simulink library "lib_feed_foward_current_control"  (R2023a)
settings: Solver=VariableStepAuto  StartTime=0.0  StopTime=10.0  RelTol=1e-3
undefined symbols (not defined in the file): parDirCurrMaxVal, parDirIndcMaxVal, parElctSpdMaxVal, parPermMagFluxMaxVal, parPhsRstnMaxVal, parQdrtCurrMaxVal, parQdrtIndcMaxVal
libraries: lib_conversion x10, lib_dynamic_saturator x2
settings Model: Creator=cav2ofo  LastModifiedBy=lenovo
settings OptimizationCC: ReuseModelBlockBuffer=off

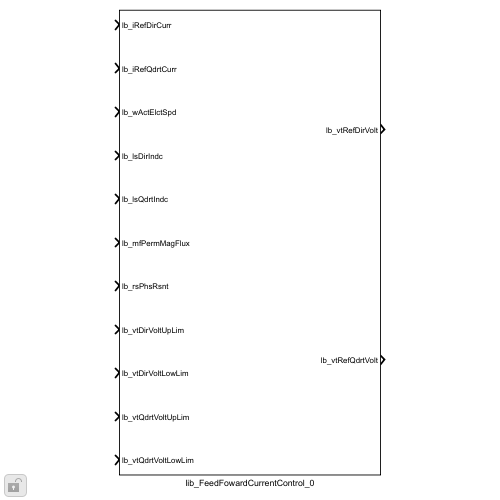
[thumbnail: Simulink's stored preview of the top-level diagram]
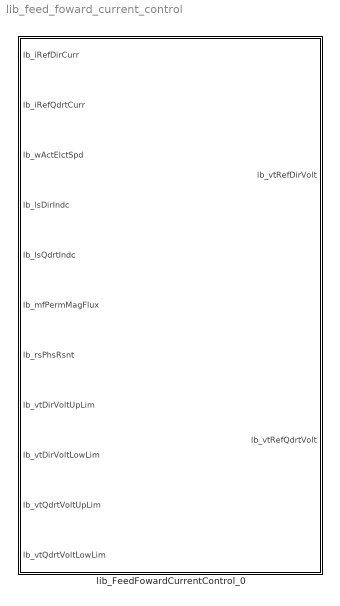
== system lib_feed_foward_current_control ==
  lib_FeedFowardCurrentControl_0 : Subsystem  mask{lb_parDirCurrMaxVal=parDirCurrMaxVal, lb_parDirCurrMinVal=-parDirCurrMaxVal, lb_parQdrtCurrMaxVal=parQdrtCurrMaxVal, lb_parQdrtCurrMinVal=-parQdrtCurrMaxVal, lb_parElctSpdMaxVal=parElctSpdMaxVal, lb_parElctSpdMinVal=-parElctSpdMaxVal, lb_parDirIndcMaxVal=parDirIndcMaxVal, lb_parQdrtIndcMaxVal=parQdrtIndcMaxVal, lb_parPhsRsntMaxVal=parPhsRstnMaxVal, lb_parPermMagFluxMaxVal=parPermMagFluxMaxVal, lb_parOutpDataType=fixdt(1,16,2^-9,0)}
      mask prompts: lb_parDirCurrMaxVal "Maximum direct current [A]:"; lb_parDirCurrMinVal "Minimum direct current [A]:"; lb_parQdrtCurrMaxVal "Maximum quadrature current [A]:"; lb_parQdrtCurrMinVal "Minimum quadrature current [A]:"; lb_parElctSpdMaxVal "Maximum electric speed [rad/s]:"; lb_parElctSpdMinVal "Minimum electric speed [rad/s]:"; lb_parDirIndcMaxVal "Maximum direct inductance [H]:"; lb_parQdrtIndcMaxVal "Maximum quadrature inductance [H]:"; lb_parPhsRsntMaxVal "Maximum phase resistance [Ohm]:"; lb_parPermMagFluxMaxVal "Maximum permanent magnet flux [Wb]:"; lb_parOutpDataType "Output data type:"
      mask init:
      | %% Req. XXX_ Define data type for product w*Lq
      | lb_parCnst1MaxVal = max(abs([lb_parElctSpdMaxVal,lb_parElctSpdMinVal]))*lb_parQdrtIndcMaxVal;
      | lb_parCnst1DataType = Simulink.NumericType;
      | lb_parCnst1DataType.DataTypeMode= 'Fixed-point: unspecified scaling';
      | lb_parCnst1DataType.Signedness = 'Signed';
      | lb_parCnst1DataType.WordLength = 16;
      | 
      | %% Req. XXX_ Define data type for product Id*Rs
      | lb_parCnst2MaxVal = max(abs([lb_parDirCurrMaxVal,lb_parDirCurrMinVal]))*lb_parPhsRsntMaxVal;
      | lb_parCnst2DataType = Simulink.NumericType;
      | lb_parCnst2DataType.DataTypeMode= 'Fixed-point: unspecified scaling';
      | lb_parCnst2DataType.Signedness = 'Signed';
      | lb_parCnst2DataType.WordLength = 16;
      | 
      | %% Req. XXX_ Define data type for product w*Lq*Iq
      | lb_parCnst3MaxVal = max(abs([lb_parQdrtCurrMaxVal,lb_parQdrtCurrMinVal]))*lb_parCnst1MaxVal;
      | lb_parCnst3DataType = Simulink.NumericType;
      | lb_parCnst3DataType.DataTypeMode= 'Fixed-point: unspecified scaling';
      | lb_parCnst3DataType.Signedness = 'Signed';
      | lb_parCnst3DataType.WordLength = 16;
      | 
      | %% Req. XXX_ Define data type for product Iq*Rs
      | lb_parCnst4MaxVal = max(abs([lb_parQdrtCurrMaxVal,lb_parQdrtCurrMinVal]))*lb_parPhsRsntMaxVal;
      | lb_parCnst4DataType = Simulink.NumericType;
      | lb_parCnst4DataType.DataTypeMode= 'Fixed-point: unspecified scaling';
      | lb_parCnst4DataType.Signedness = 'Signed';
      | lb_parCnst4DataType.WordLength = 16;
      | 
      | %% Req. XXX_ Define data type for product w*Ld
      | lb_parCnst5MaxVal = max(abs([lb_parElctSpdMaxVal,lb_parElctSpdMinVal]))*lb_parDirIndcMaxVal;
      | lb_parCnst5DataType = Simulink.NumericType;
      | lb_parCnst5DataType.DataTypeMode= 'Fixed-point: unspecified scaling';
      | lb_parCnst5DataType.Signedness = 'Signed';
      | lb_parCnst5DataType.WordLength = 16;
      | 
      | %% Req. XXX_ Define data type for product w*Ld*Id
      | lb_parCnst6MaxVal = max(abs([lb_parDirCurrMaxVal,lb_parDirCurrMinVal]))*lb_parCnst5MaxVal;
      | lb_parCnst6DataType = Simulink.NumericType;
      | lb_parCnst6DataType.DataTypeMode= 'Fixed-point: unspecified scaling';
      | lb_parCnst6DataType.Signedness = 'Signed';
      | lb_parCnst6DataType.WordLength = 16;
      | 
      | %% Req. XXX_ Define data type for product Iq*Rs+w*Ld*Id
      | lb_parCnst7MaxVal = lb_parCnst4MaxVal+lb_parCnst6MaxVal;
      | lb_parCnst7DataType = Simulink.NumericType;
      | lb_parCnst7DataType.DataTypeMode= 'Fixed-point: unspecified scaling';
      | lb_parCnst7DataType.Signedness = 'Signed';
      | lb_parCnst7DataType.WordLength = 16;
      | 
      | %% Req. XXX_ Define data type for product w*Ld
      | lb_parCnst8MaxVal = max(abs([lb_parElctSpdMaxVal,lb_parElctSpdMinVal]))*lb_parPermMagFluxMaxVal;
      | lb_parCnst8DataType = Simulink.NumericType;
      | lb_parCnst8DataType.DataTypeMode= 'Fixed-point: unspecified scaling';
      | lb_parCnst8DataType.Signedness = 'Signed';
      | lb_parCnst8DataType.WordLength = 16;
      mask TypeOptions lb_parOutpDataType: sss_DirectCurrentCoupling/lib_Conversion_1/lb_parDataType | sss_QuadratureCurrentCoupling/lib_Conversion_1/lb_parDataType
      mask DialogControl DescGroupVar Prompt: Current Coupling block
      mask DialogControl DescTextVar Prompt: This block computes the direct and quadrature voltage references.
      mask DialogControl modlPar Prompt: Parameter
      mask DialogControl Container3 Prompt: Data type

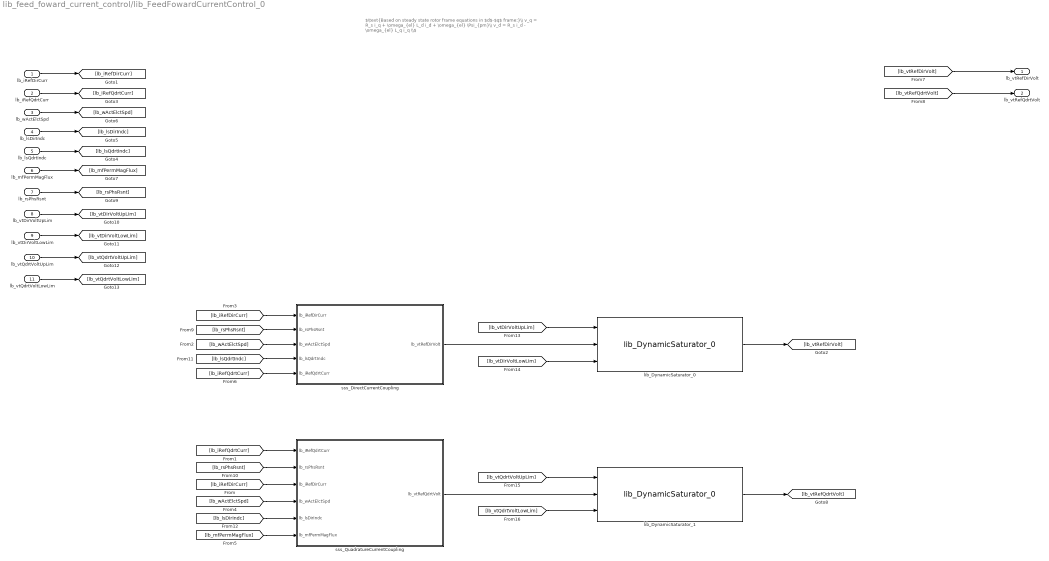
== system lib_feed_foward_current_control/lib_FeedFowardCurrentControl_0 ==
  note: $\text{Based on steady state rotor frame equations in $d$-$q$ frame:}\\ v_q = R_s i_q + \omega_{el} L_d i_d + \omega_{el} \Psi_{pm}\\ v_d = R_s i_d - \omega_{el} L_q i_q \\$
  lb_iRefDirCurr : Inport
  lb_iRefQdrtCurr : Inport  Port=2
  lb_wActElctSpd : Inport  Port=3
  lb_lsDirIndc : Inport  Port=4
  lb_lsQdrtIndc : Inport  Port=5
  lb_mfPermMagFlux : Inport  Port=6
  lb_rsPhsRsnt : Inport  Port=7
  lb_vtDirVoltUpLim : Inport  Port=8
  lb_vtDirVoltLowLim : Inport  Port=9
  lb_vtQdrtVoltUpLim : Inport  Port=10
  lb_vtQdrtVoltLowLim : Inport  Port=11
  lib_DynamicSaturator_0 : lib_dynamic_saturator/lib_DynamicSaturator_0
  lib_DynamicSaturator_1 : lib_dynamic_saturator/lib_DynamicSaturator_0
  sss_DirectCurrentCoupling : Subsystem
  sss_QuadratureCurrentCoupling : Subsystem
  lb_vtRefDirVolt : Outport
  lb_vtRefQdrtVolt : Outport  Port=2
  wires:
  [lb_wActElctSpd] -> sss_QuadratureCurrentCoupling/4(lb_wActElctSpd)
  lb_iRefDirCurr/1 -> [lb_iRefDirCurr]
  [lb_iRefDirCurr] -> sss_DirectCurrentCoupling/1(lb_iRefDirCurr)
  lb_lsDirIndc/1 -> [lb_lsDirIndc]
  [lb_vtRefQdrtVolt] -> lb_vtRefQdrtVolt/1
  [lb_wActElctSpd] -> sss_DirectCurrentCoupling/3(lb_wActElctSpd)
  lb_iRefQdrtCurr/1 -> [lb_iRefQdrtCurr]
  lb_lsQdrtIndc/1 -> [lb_lsQdrtIndc]
  [lb_mfPermMagFlux] -> sss_QuadratureCurrentCoupling/6(lb_mfPermMagFlux)
  [lb_iRefQdrtCurr] -> sss_DirectCurrentCoupling/5(lb_iRefQdrtCurr)
  lb_wActElctSpd/1 -> [lb_wActElctSpd]
  [lb_vtRefDirVolt] -> lb_vtRefDirVolt/1
  lb_mfPermMagFlux/1 -> [lb_mfPermMagFlux]
  [lb_iRefQdrtCurr] -> sss_QuadratureCurrentCoupling/1(lb_iRefQdrtCurr)
  [lb_iRefDirCurr] -> sss_QuadratureCurrentCoupling/3(lb_iRefDirCurr)
  lb_rsPhsRsnt/1 -> [lb_rsPhsRsnt]
  [lb_rsPhsRsnt] -> sss_DirectCurrentCoupling/2(lb_rsPhsRsnt)
  [lb_rsPhsRsnt] -> sss_QuadratureCurrentCoupling/2(lb_rsPhsRsnt)
  lib_DynamicSaturator_0/1 -> [lb_vtRefDirVolt]
  [lb_vtDirVoltUpLim] -> lib_DynamicSaturator_0/1
  [lb_vtDirVoltLowLim] -> lib_DynamicSaturator_0/3
  lib_DynamicSaturator_1/1 -> [lb_vtRefQdrtVolt]
  [lb_vtQdrtVoltLowLim] -> lib_DynamicSaturator_1/3
  [lb_vtQdrtVoltUpLim] -> lib_DynamicSaturator_1/1
  [lb_lsQdrtIndc] -> sss_DirectCurrentCoupling/4(lb_lsQdrtIndc)
  [lb_lsDirIndc] -> sss_QuadratureCurrentCoupling/5(lb_lsDirIndc)
  sss_DirectCurrentCoupling/1(lb_vtRefDirVolt) -> lib_DynamicSaturator_0/2
  sss_QuadratureCurrentCoupling/1(lb_vtRefQdrtVolt) -> lib_DynamicSaturator_1/2
  lb_vtDirVoltUpLim/1 -> [lb_vtDirVoltUpLim]
  lb_vtDirVoltLowLim/1 -> [lb_vtDirVoltLowLim]
  lb_vtQdrtVoltUpLim/1 -> [lb_vtQdrtVoltUpLim]
  lb_vtQdrtVoltLowLim/1 -> [lb_vtQdrtVoltLowLim]

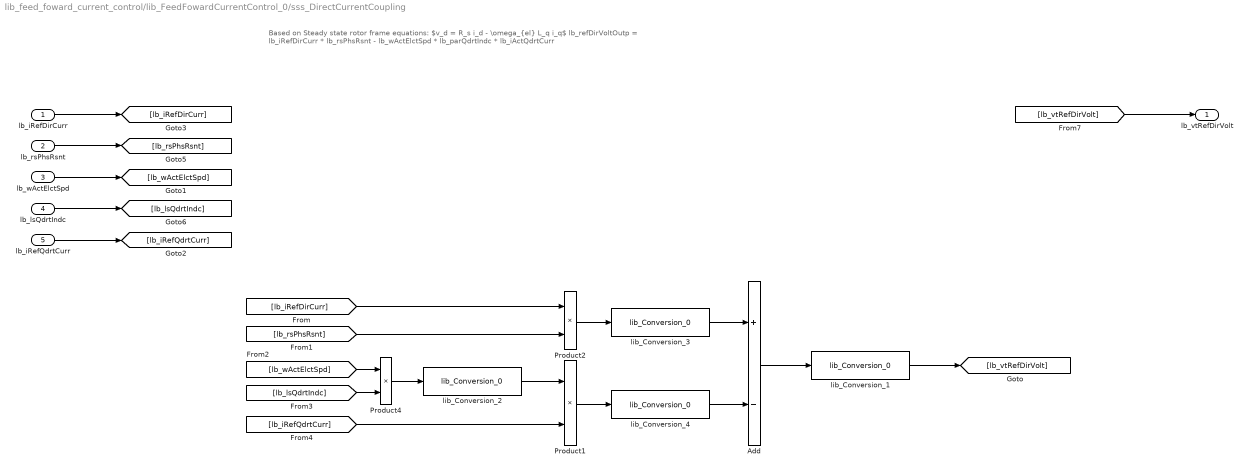
== system lib_feed_foward_current_control/lib_FeedFowardCurrentControl_0/sss_DirectCurrentCoupling ==
  note: Based on Steady state rotor frame equations:
      | $v_d = R_s i_d - \omega_{el} L_q i_q$
      | lb_refDirVoltOutp = lb_iRefDirCurr * lb_rsPhsRsnt
      | - lb_wActElctSpd * lb_parQdrtIndc * lb_iActQdrtCurr
  lb_iRefDirCurr : Inport
  lb_rsPhsRsnt : Inport  Port=2
  lb_wActElctSpd : Inport  Port=3
  lb_lsQdrtIndc : Inport  Port=4
  lb_iRefQdrtCurr : Inport  Port=5
  Add : Sum  Inputs=+-  OutDataTypeStr=Inherit: Inherit via back propagation  RndMeth=Simplest
  Product1 : Product  OutDataTypeStr=Inherit: Inherit via back propagation  RndMeth=Simplest
  Product2 : Product  OutDataTypeStr=Inherit: Inherit via back propagation  RndMeth=Simplest
  Product4 : Product  OutDataTypeStr=Inherit: Inherit via back propagation  RndMeth=Simplest
  lib_Conversion_1 : lib_conversion/lib_Conversion_0  lb_parDataType=fixdt(1,16,2^-9,0)  lb_parOutpMaxVal=[]  lb_parOutpMinVal=[]  lb_parSatFlag=off
  lib_Conversion_2 : lib_conversion/lib_Conversion_0  lb_parDataType=lb_parCnst1DataType  lb_parOutpMaxVal=lb_parCnst1MaxVal  lb_parOutpMinVal=[]  lb_parSatFlag=off
  lib_Conversion_3 : lib_conversion/lib_Conversion_0  lb_parDataType=lb_parCnst2DataType  lb_parOutpMaxVal=lb_parCnst2MaxVal  lb_parOutpMinVal=[]  lb_parSatFlag=off
  lib_Conversion_4 : lib_conversion/lib_Conversion_0  lb_parDataType=lb_parCnst3DataType  lb_parOutpMaxVal=lb_parCnst3MaxVal  lb_parOutpMinVal=[]  lb_parSatFlag=off
  lb_vtRefDirVolt : Outport
  wires:
  Add/1 -> lib_Conversion_1/1
  Product1/1 -> lib_Conversion_4/1
  Product4/1 -> lib_Conversion_2/1
  lib_Conversion_2/1 -> Product1/1
  lib_Conversion_4/1 -> Add/2
  Product2/1 -> lib_Conversion_3/1
  lib_Conversion_3/1 -> Add/1
  [lb_vtRefDirVolt] -> lb_vtRefDirVolt/1
  lib_Conversion_1/1 -> [lb_vtRefDirVolt]
  lb_iRefDirCurr/1 -> [lb_iRefDirCurr]
  [lb_iRefDirCurr] -> Product2/1
  lb_rsPhsRsnt/1 -> [lb_rsPhsRsnt]
  [lb_rsPhsRsnt] -> Product2/2
  lb_wActElctSpd/1 -> [lb_wActElctSpd]
  [lb_wActElctSpd] -> Product4/1
  [lb_lsQdrtIndc] -> Product4/2
  lb_lsQdrtIndc/1 -> [lb_lsQdrtIndc]
  lb_iRefQdrtCurr/1 -> [lb_iRefQdrtCurr]
  [lb_iRefQdrtCurr] -> Product1/2

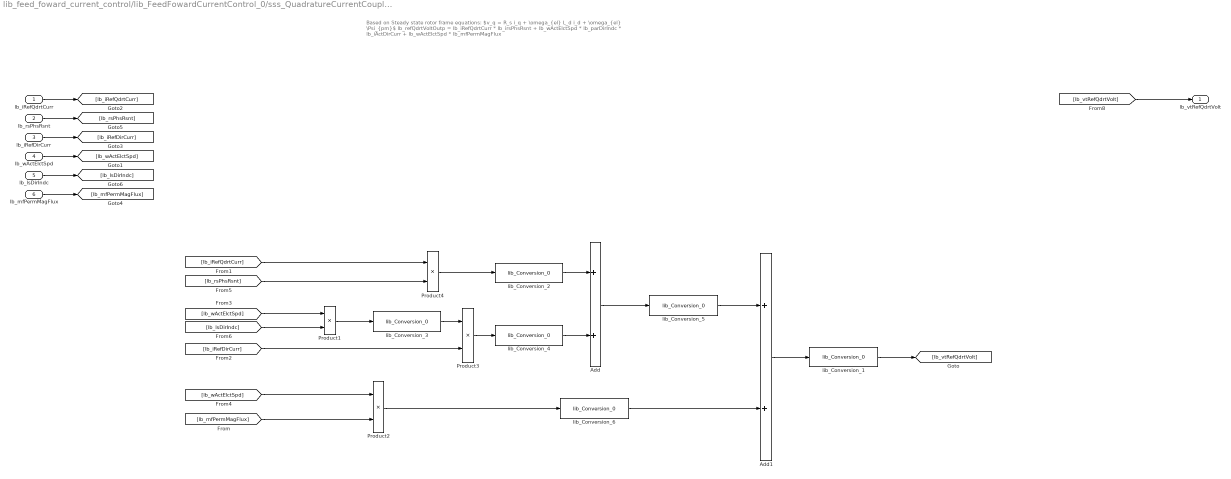
== system lib_feed_foward_current_control/lib_FeedFowardCurrentControl_0/sss_QuadratureCurrentCoupling ==
  note: Based on Steady state rotor frame equations:
      | $v_q = R_s i_q + \omega_{el} L_d i_d + \omega_{el} \Psi_{pm}$
      | lb_refQdrtVoltOutp = lb_iRefQdrtCurr * lb_irsPhsRsnt +
      | lb_wActElctSpd * lb_parDirIndc * lb_iActDirCurr +
      | lb_wActElctSpd * lb_mfPermMagFlux
  lb_iRefQdrtCurr : Inport
  lb_rsPhsRsnt : Inport  Port=2
  lb_iRefDirCurr : Inport  Port=3
  lb_wActElctSpd : Inport  Port=4
  lb_lsDirIndc : Inport  Port=5
  lb_mfPermMagFlux : Inport  Port=6
  Add : Sum  OutDataTypeStr=Inherit: Inherit via back propagation  RndMeth=Simplest
  Add1 : Sum  OutDataTypeStr=Inherit: Inherit via back propagation  RndMeth=Simplest
  Product{1..4} (4 alike) : Product  OutDataTypeStr=Inherit: Inherit via back propagation  RndMeth=Simplest
  lib_Conversion_1 : lib_conversion/lib_Conversion_0  lb_parDataType=fixdt(1,16,2^-9,0)  lb_parOutpMaxVal=[]  lb_parOutpMinVal=[]  lb_parSatFlag=off
  lib_Conversion_2 : lib_conversion/lib_Conversion_0  lb_parDataType=lb_parCnst4DataType  lb_parOutpMaxVal=lb_parCnst4MaxVal  lb_parOutpMinVal=[]  lb_parSatFlag=off
  lib_Conversion_3 : lib_conversion/lib_Conversion_0  lb_parDataType=lb_parCnst5DataType  lb_parOutpMaxVal=lb_parCnst5MaxVal  lb_parOutpMinVal=[]  lb_parSatFlag=off
  lib_Conversion_4 : lib_conversion/lib_Conversion_0  lb_parDataType=lb_parCnst6DataType  lb_parOutpMaxVal=lb_parCnst6MaxVal  lb_parOutpMinVal=[]  lb_parSatFlag=off
  lib_Conversion_5 : lib_conversion/lib_Conversion_0  lb_parDataType=lb_parCnst7DataType  lb_parOutpMaxVal=lb_parCnst7MaxVal  lb_parOutpMinVal=[]  lb_parSatFlag=off
  lib_Conversion_6 : lib_conversion/lib_Conversion_0  lb_parDataType=lb_parCnst8DataType  lb_parOutpMaxVal=lb_parCnst8MaxVal  lb_parOutpMinVal=[]  lb_parSatFlag=off
  lb_vtRefQdrtVolt : Outport
  wires:
  Add1/1 -> lib_Conversion_1/1
  lb_iRefQdrtCurr/1 -> [lb_iRefQdrtCurr]
  lb_iRefDirCurr/1 -> [lb_iRefDirCurr]
  lb_wActElctSpd/1 -> [lb_wActElctSpd]
  lb_mfPermMagFlux/1 -> [lb_mfPermMagFlux]
  [lb_mfPermMagFlux] -> Product2/2
  [lb_wActElctSpd] -> Product2/1
  [lb_lsDirIndc] -> Product1/2
  Product1/1 -> lib_Conversion_3/1
  [lb_iRefDirCurr] -> Product3/2
  [lb_wActElctSpd] -> Product1/1
  lib_Conversion_3/1 -> Product3/1
  Product3/1 -> lib_Conversion_4/1
  lib_Conversion_4/1 -> Add/2
  Add/1 -> lib_Conversion_5/1
  lib_Conversion_5/1 -> Add1/1
  Product2/1 -> lib_Conversion_6/1
  lib_Conversion_6/1 -> Add1/2
  lb_rsPhsRsnt/1 -> [lb_rsPhsRsnt]
  Product4/1 -> lib_Conversion_2/1
  [lb_iRefQdrtCurr] -> Product4/1
  [lb_rsPhsRsnt] -> Product4/2
  lb_lsDirIndc/1 -> [lb_lsDirIndc]
  lib_Conversion_2/1 -> Add/1
  [lb_vtRefQdrtVolt] -> lb_vtRefQdrtVolt/1
  lib_Conversion_1/1 -> [lb_vtRefQdrtVolt]
